simulink model "robot_try"  (R2023a)
settings: Solver=VariableStepAuto  StartTime=0.0  StopTime=10  RelTol=1e-3
undefined symbols (not defined in the file): L, Ts
settings Model: Creator=raulD  LastModifiedBy=raulD

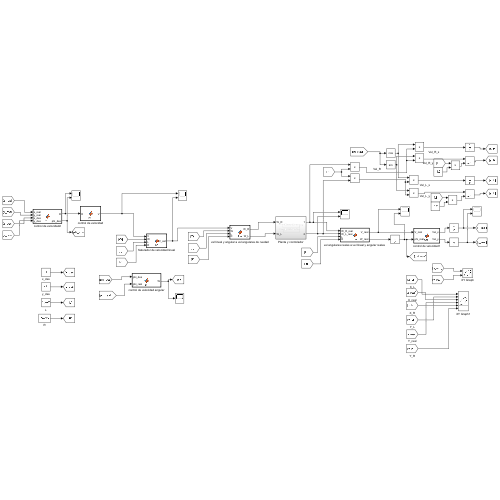
[thumbnail: Simulink's stored preview of the top-level diagram]
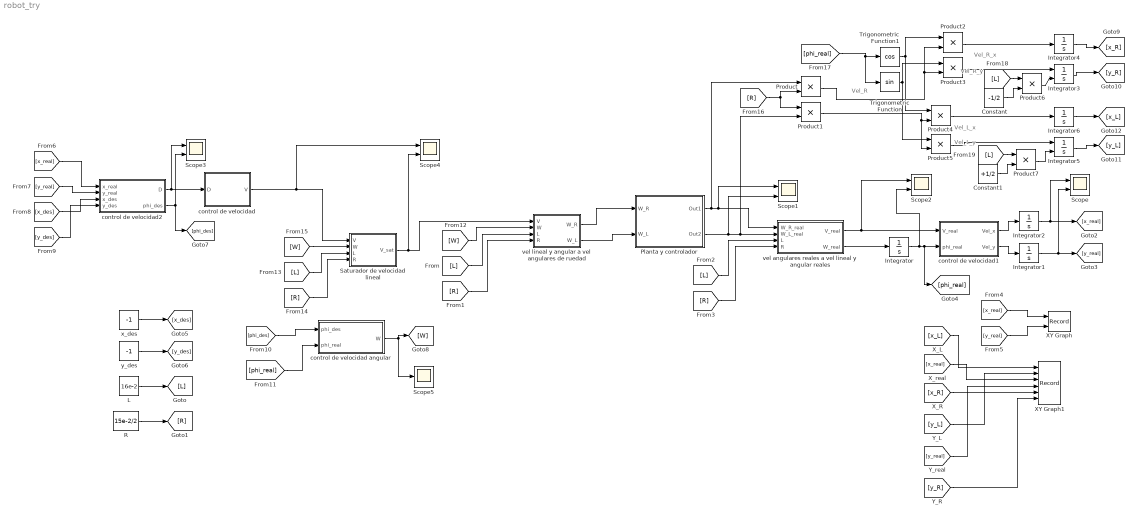
== system robot_try ==
  note: Vel_R_y
  note: Vel_R
  note: Vel_R_x
  note: Vel_L_y
  note: Vel_L_x
  Constant : Constant  Value=-1/2
  Constant1 : Constant  Value=+1/2
  Integrator : Integrator  ContinuousStateAttributes='phi'
  Integrator1 : Integrator  ContinuousStateAttributes='y'
  Integrator2 : Integrator  ContinuousStateAttributes='x'
  Integrator3 : Integrator  InitialConditionSource=external  InitialCondition=-L/2  ContinuousStateAttributes='y'
  Integrator4 : Integrator  ContinuousStateAttributes='x'
  Integrator5 : Integrator  InitialConditionSource=external  ContinuousStateAttributes='y'
  Integrator6 : Integrator  ContinuousStateAttributes='x'
  L : Constant  Value=16e-2
  Planta y controlador : Subsystem
  Product{,1..7} (8 alike) : Product
  R : Constant  Value=15e-2/2
  Saturador de velocidad lineal : MATLAB Function  TreatAsAtomicUnit=on
  Scope{,1..4} (5 alike) : Scope  NumInputPorts=2
  Scope5 : Scope
  Trigonometric Function : Trigonometry
  Trigonometric Function1 : Trigonometry  Operator=cos
  XY Graph : Record  FileSettingsInternal="{\"entries\":[{\"content\":{\"excelSettings\":{\"content\":{},\"type\":\"Streamout.ExcelSettings\"}},\"type\":\"Streamout.FileSettingStorage\",\"uuid\":\"\"}],\"packageUris\":[\"http:\\/\\/schema.mathworks.com\\/mf0\\/streamout_blocks\\/R2020a\"],\"version\":\"1.0\"}"  Layout=[1 1]  SignalsInternal="{\"entries\":[{\"content\":{\"signals\":[{\"content\":{\"blockPath\":[],\"dimensions\":[1],\"domain\":\"\",\"lineColor\":\"#a2142f\",\"plots\":[1],\"port\":1,\"sid\":[\"\"],\"signalID\":1467,\"signalName\":\"From4\"},\"type\":\"RecordBlkView.Signal\",\"uuid\":\"\"},{\"content\":{\"blockPath\":[],\"dimensions\":[1],\"domain\":\"\",\"lineColor\":\"#139fff\",\"plots\":[1],\"port\":2,\"sid\":[\"\"],\"signalID\":1471,\"signalName\":\"From5\"},\"type\":\"RecordBlkView.Signal\",\"uuid\":\"\"}]},\"type\":\"RecordBlkView.InputSignals\",\"uuid\":\"\"}],\"packageUris\":[\"http:\\/\\/schema.mathworks.com\\/mf0\\/streamout_blocks\\/R2020a\"],\"version\":\"1.0\"}"  VisualizationBindings="{\"xyplotplugin\":{\"info\":[{\"series\":[{\"bindingParametersList\":[{\"parameter\":\"X-Axis\",\"signalID\":1467,\"signalName\":\"From4\"},{\"parameter\":\"Y-Axis\",\"signalID\":1471,\"signalName\":\"From5\"}],\"seriesID\":51917}],\"subplotID\":1}]}}"  CompatibilityTag=XY
  XY Graph1 : Record  FileSettingsInternal="{\"entries\":[{\"content\":{\"excelSettings\":{\"content\":{},\"type\":\"Streamout.ExcelSettings\"}},\"type\":\"Streamout.FileSettingStorage\",\"uuid\":\"\"}],\"packageUris\":[\"http:\\/\\/schema.mathworks.com\\/mf0\\/streamout_blocks\\/R2020a\"],\"version\":\"1.0\"}"  Layout=[1 1]  SignalsInternal="{\"entries\":[{\"content\":{\"signals\":[{\"content\":{\"blockPath\":[],\"dimensions\":[1],\"domain\":\"\",\"lineColor\":\"#a2142f\",\"port\":1,\"sid\":[\"\"],\"signalID\":1475,\"signalName\":\"X_L\"},\"type\":\"RecordBlkView.Signal\",\"uuid\":\"\"},{\"content\":{\"blockPath\":[],\"dimensions\":[1],\"domain\":\"\",\"lineColor\":\"#139fff\",\"port\":2,\"sid\":[\"\"],\"signalID\":1479,\"signalName\":\"Y_L\"},\"type\":\"RecordBlkView.Signal\",\"uuid\":\"\"},{\"content\":{\"blockPath\":[],\"dimensions\":[1],\"domain\":\"\",\"lineColor\":\"#a2142f\",\"port\":3,\"sid\":[\"\"],\"signalID\":1483,\"signalName\":\"X_real\"},\"type\":\"RecordBlkView.Signal\",\"uuid\":\"\"},{\"content\":{\"blockPath\":[],\"dimensions\":[1],\"domain\":\"\",\"lineColor\":\"#139fff\",\"port\":4,\"sid\":[\"\"],\"signalID\":1487,\"signalName\":\"Y_real\"},\"type\":\"RecordBlkView.Signal\",\"uuid\":\"\"},{\"content\":{\"blockPath\":[],\"dimensions\":[1],\"domain\":\"\",\"lineColor\":\"#ff6929\",\"port\":5,\"sid\":[\"\"],\"signalID\":1491,\"signalName\":\"X_R\"},\"type\":\"RecordBlkView.Signal\",\"uuid\":\"\"},{\"content\":{\"blockPath\":[],\"dimensions\":[1],\"domain\":\"\",\"lineColor\":\"#b746ff\",\"port\":6,\"sid\":[\"\"],\"signalID\":1495,\"signalName\":\"Y_R\"},\"type\":\"RecordBlkView.Signal\",\"uuid\":\"\"}]},\"type\":\"RecordBlkView.InputSignals\",\"uuid\":\"\"}],\"packageUris\":[\"http:\\/\\/schema.mathworks.com\\/mf0\\/streamout_blocks\\/R2020a\"],\"version\":\"1.0\"}"  VisualizationBindings="{\"xyplotplugin\":{\"info\":[{\"series\":[],\"subplotID\":1}]}}"  CompatibilityTag=XY
  control de velocidad : MATLAB Function  TreatAsAtomicUnit=on
  control de velocidad angular : MATLAB Function  TreatAsAtomicUnit=on
  control de velocidad1 : MATLAB Function  TreatAsAtomicUnit=on
  control de velocidad2 : MATLAB Function  TreatAsAtomicUnit=on
  "vel angulares reales a vel lineal y angular reales " : MATLAB Function  TreatAsAtomicUnit=on
  vel lineal y angular a vel angulares de ruedad : MATLAB Function  TreatAsAtomicUnit=on
  x_des : Constant  Value=-1
  y_des : Constant  Value=-1
  wires:
  L/1 -> [L]
  [L] -> vel lineal y angular a vel angulares de ruedad/3(L)
  R/1 -> [R]
  [R] -> vel lineal y angular a vel angulares de ruedad/4(R)
  vel lineal y angular a vel angulares de ruedad/1(W_R) -> Planta y controlador/1(W_R)
  vel lineal y angular a vel angulares de ruedad/2(W_L) -> Planta y controlador/2(W_L)
  control de velocidad/1(V) -> Scope4/1, Saturador de velocidad lineal/1(V)
  [L] -> "vel angulares reales a vel lineal y angular reales "/3(L)
  [R] -> "vel angulares reales a vel lineal y angular reales "/4(R)
  Planta y controlador/1(Out1) -> Product/1, Scope1/1, "vel angulares reales a vel lineal y angular reales "/1(W_R_real)
  Planta y controlador/2(Out2) -> Scope1/2, Product1/2, "vel angulares reales a vel lineal y angular reales "/2(W_L_real)
  "vel angulares reales a vel lineal y angular reales "/2(W_real) -> Integrator/1
  Integrator/1 -> Scope2/2, [phi_real], control de velocidad1/2(phi_real)
  "vel angulares reales a vel lineal y angular reales "/1(V_real) -> Scope2/1, control de velocidad1/1(V_real)
  control de velocidad1/2(Vel_y) -> Integrator1/1
  control de velocidad1/1(Vel_x) -> Integrator2/1
  Integrator2/1 -> Scope/1, [x_real]
  Integrator1/1 -> Scope/2, [y_real]
  [y_real] -> XY Graph/2
  [x_real] -> XY Graph/1
  x_des/1 -> [x_des]
  y_des/1 -> [y_des]
  [x_real] -> control de velocidad2/1(x_real)
  [y_real] -> control de velocidad2/2(y_real)
  [x_des] -> control de velocidad2/3(x_des)
  [y_des] -> control de velocidad2/4(y_des)
  control de velocidad2/2(phi_des) -> Scope3/2, [phi_des]
  [W] -> vel lineal y angular a vel angulares de ruedad/2(W)
  control de velocidad2/1(D) -> Scope3/1, control de velocidad/1(D)
  [L] -> Saturador de velocidad lineal/3(L)
  [W] -> Saturador de velocidad lineal/2(W)
  [R] -> Saturador de velocidad lineal/4(R)
  Saturador de velocidad lineal/1(V_sat) -> Scope4/2, vel lineal y angular a vel angulares de ruedad/1(V)
  [R] -> Product/2, Product1/1
  [phi_real] -> Trigonometric Function/1, Trigonometric Function1/1
  Trigonometric Function1/1 -> Product2/1, Product4/1
  Product/1 -> Product2/2, Product3/2
  Trigonometric Function/1 -> Product5/1, Product3/1
  Product2/1 -> Integrator4/1
  Product3/1 -> Integrator3/1
  Integrator3/1 -> [y_R]
  Integrator4/1 -> [x_R]
  Integrator6/1 -> [x_L]
  Integrator5/1 -> [y_L]
  Product5/1 -> Integrator5/1
  Product4/1 -> Integrator6/1
  Product1/1 -> Product5/2, Product4/2
  [L] -> Product6/1
  Constant/1 -> Product6/2
  Product6/1 -> Integrator3/2
  Product7/1 -> Integrator5/2
  Constant1/1 -> Product7/2
  [L] -> Product7/1
  [x_L] -> XY Graph1/1
  [y_L] -> XY Graph1/2
  [x_real] -> XY Graph1/3
  [y_real] -> XY Graph1/4
  [x_R] -> XY Graph1/5
  [y_R] -> XY Graph1/6
  [phi_des] -> control de velocidad angular/1(phi_des)
  [phi_real] -> control de velocidad angular/2(phi_real)
  control de velocidad angular/1(W) -> [W], Scope5/1

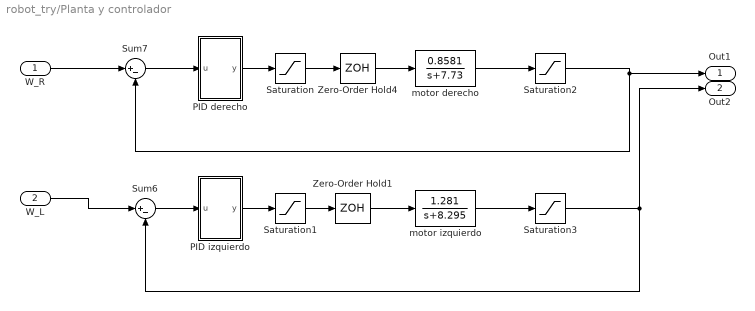
== system robot_try/Planta y controlador ==
  W_R : Inport
  W_L : Inport  Port=2
  PID derecho : Subsystem
  PID izquierdo : Subsystem
  Saturation : Saturate  UpperLimit=100  LowerLimit=-100
  Saturation1 : Saturate  UpperLimit=100  LowerLimit=-100
  Saturation2 : Saturate  UpperLimit=11  LowerLimit=-11
  Saturation3 : Saturate  UpperLimit=11  LowerLimit=-11
  Sum6 : Sum  Inputs=|+-
  Sum7 : Sum  Inputs=|+-
  Zero-Order Hold1 : ZeroOrderHold  SampleTime=Ts
  Zero-Order Hold4 : ZeroOrderHold  SampleTime=Ts
  motor derecho : TransferFcn  Numerator=[0.8581]  Denominator=[1 7.73]
  motor izquierdo : TransferFcn  Numerator=[1.281]  Denominator=[1 8.295]
  Out1 : Outport
  Out2 : Outport  Port=2
  wires:
  W_L/1 -> Sum6/1
  Zero-Order Hold1/1 -> motor izquierdo/1
  W_R/1 -> Sum7/1
  Zero-Order Hold4/1 -> motor derecho/1
  Sum6/1 -> PID izquierdo/1(u)
  Sum7/1 -> PID derecho/1(u)
  Saturation/1 -> Zero-Order Hold4/1
  PID derecho/1(y) -> Saturation/1
  PID izquierdo/1(y) -> Saturation1/1
  Saturation1/1 -> Zero-Order Hold1/1
  motor derecho/1 -> Saturation2/1
  motor izquierdo/1 -> Saturation3/1
  Saturation2/1 -> Out1/1, Sum7/2
  Saturation3/1 -> Out2/1, Sum6/2

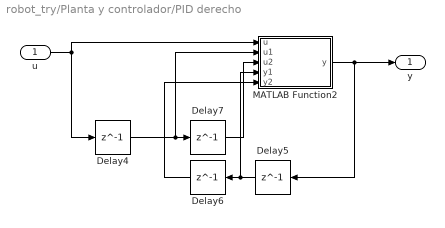
== system robot_try/Planta y controlador/PID derecho ==
  u : Inport
  Delay{4..7} (4 alike) : Delay  DelayLength=1  InitialCondition=0  SampleTime=Ts
  MATLAB Function2 : MATLAB Function  TreatAsAtomicUnit=on
  y : Outport
  wires:
  MATLAB Function2/1(y) -> Delay5/1, y/1
  u/1 -> MATLAB Function2/1(u), Delay4/1
  Delay6/1 -> MATLAB Function2/5(y2)
  Delay7/1 -> MATLAB Function2/3(u2)
  Delay4/1 -> Delay7/1, MATLAB Function2/2(u1)
  Delay5/1 -> Delay6/1, MATLAB Function2/4(y1)

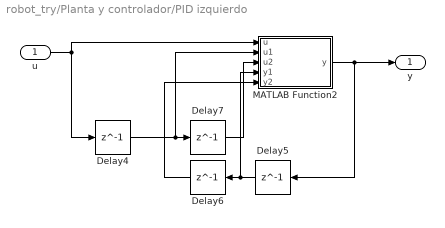
== system robot_try/Planta y controlador/PID izquierdo ==
  u : Inport
  Delay{4..7} (4 alike) : Delay  DelayLength=1  InitialCondition=0  SampleTime=Ts
  MATLAB Function2 : MATLAB Function  TreatAsAtomicUnit=on
  y : Outport
  wires:
  Delay5/1 -> MATLAB Function2/4(y1), Delay6/1
  Delay4/1 -> MATLAB Function2/2(u1), Delay7/1
  Delay7/1 -> MATLAB Function2/3(u2)
  Delay6/1 -> MATLAB Function2/5(y2)
  u/1 -> Delay4/1, MATLAB Function2/1(u)
  MATLAB Function2/1(y) -> y/1, Delay5/1

== matlab function robot_try/Planta y controlador/PID izquierdo/MATLAB Function2 ==
  data: u input; y output; u1 input; u2 input; y1 input; y2 input
function y = fcn(u, u1, u2, y1, y2)

y = 13.28*u-6.997*u1-4.867*u2+0.9404*y1+0.05964*y2;

== matlab function robot_try/vel lineal y angular a vel angulares de ruedad ==
  data: V input; W_R output; W input; L input; R input; W_L output
function [W_R,W_L] = fcn(V,W,L,R)

V_R = V+W*L/2;
V_L = V-W*L/2;

W_R = V_R/R;
W_L = V_L/R;

== matlab function robot_try/control de velocidad ==
  data: D input; V output
function V = fcn(D)

P = 0.5;
V = P*D;

== matlab function robot_try/Planta y controlador/PID derecho/MATLAB Function2 ==
  data: u input; y output; u1 input; u2 input; y1 input; y2 input
function y = fcn(u, u1, u2, y1, y2)

y = 15.99*u-6.576*u1-7.715*u2+0.9847*y1+0.01531*y2;

== matlab function robot_try/vel angulares reales a vel lineal y angular reales  ==
  data: W_R_real input; V_real output; W_L_real input; L input; R input; W_real output
function [V_real,W_real] = fcn(W_R_real,W_L_real,L,R)

V_real = ((W_R_real+W_L_real)*R)/2;
W_real = ((W_R_real-W_L_real)*R)/L;

== matlab function robot_try/control de velocidad1 ==
  data: V_real input; Vel_x output; phi_real input; Vel_y output
function [Vel_x,Vel_y] = fcn(V_real,phi_real)

Vel_x = V_real*cos(phi_real);

Vel_y = V_real*sin(phi_real);

== matlab function robot_try/control de velocidad2 ==
  data: x_real input; D output; phi_des output; y_real input; x_des input; y_des input
function [D,phi_des] = fcn(x_real,y_real,x_des,y_des)

delta_x = x_des-x_real;
delta_y = y_des-y_real;

phi_des = atan2(delta_y,delta_x);

D = (delta_x^2+delta_y^2)^(1/2);

== matlab function robot_try/Saturador de velocidad lineal ==
  data: V input; V_sat output; W input; L input; R input
function V_sat = fcn(V,W,L,R)

W_R_max = 11;
W_L_max = 11;

V_max_R = W_R_max*R-(W*L)/2;
V_max_L = W_L_max*R+(W*L)/2;

if V_max_R > V_max_L
    V_max = V_max_L;
else
    V_max = V_max_R;
end

if V_max < 0.1
    V_max = 0.1;
end

if V > V_max
    V_sat = V_max;
else
    V_sat = V;
end

== matlab function robot_try/control de velocidad angular ==
  data: phi_des input; W output; phi_real input
function W = fcn(phi_des, phi_real)

error = phi_des-phi_real;
P = 10;

W = error*P;
